simulink library "cdsRampSwitch"  (Simulink 6.2)
settings Model: LastModifiedBy=rolf

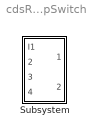
== system cdsRampSwitch ==
  Subsystem : Subsystem

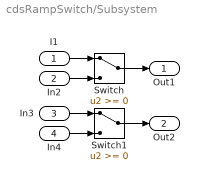
== system cdsRampSwitch/Subsystem ==
  I1 : Inport  Port=1  LatchInput=off
  In2 : Inport  Port=2  LatchInput=off
  In3 : Inport  Port=3  LatchInput=off
  In4 : Inport  Port=4  LatchInput=off
  Switch : Switch
  Switch1 : Switch
  Out1 : Outport
  Out2 : Outport  Port=2
  wires:
  I1/1 -> Switch/1
  Switch/1 -> Out1/1
  In2/1 -> Switch/3
  In3/1 -> Switch1/1
  Switch1/1 -> Out2/1
  In4/1 -> Switch1/3
